simulink model "tcp"  (R2021b)
settings: Solver=VariableStepAuto  StartTime=0.0  StopTime=inf  RelTol=1e-3
undefined symbols (not defined in the file): f
libraries: instrumentlib x4
settings Model: Creator=sdoda3  LastModifiedBy=ae-dagbeyibor3

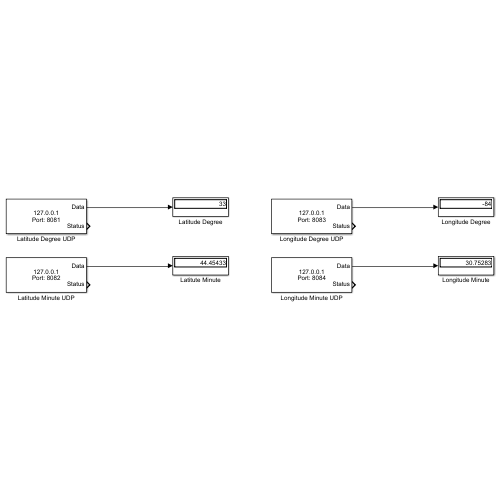
[thumbnail: Simulink's stored preview of the top-level diagram]
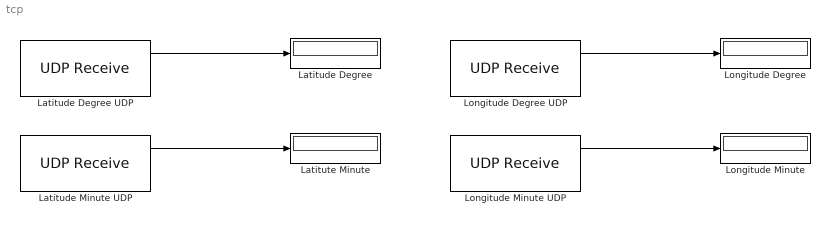
== system tcp ==
  Latitude Degree : Display
  Latitude Degree UDP : instrumentlib/UDP Receive  Priority=1  Host=127.0.0.1  Port=8081  LocalPort=8081  EnablePortSharing=off  GetLatestData=off  DataSize=[1 1]  DataType=int16  ASCIIFormatting=%f,  Terminator=LF  ByteOrder=BigEndian  EnableBlockingMode=off  Timeout=5  SampleTime=0.01  LocalAddress=127.0.0.1
  Latitude Minute UDP : instrumentlib/UDP Receive  Priority=1  Host=127.0.0.1  Port=8081  LocalPort=8082  EnablePortSharing=off  GetLatestData=off  DataSize=[1 1]  DataType=single  ASCIIFormatting=%f,  Terminator=LF  ByteOrder=BigEndian  EnableBlockingMode=off  Timeout=5  SampleTime=0.01  LocalAddress=127.0.0.1
  Latitute Minute : Display
  Longitude Degree : Display
  Longitude Degree UDP : instrumentlib/UDP Receive  Priority=1  Host=127.0.0.1  Port=8081  LocalPort=8083  EnablePortSharing=off  GetLatestData=off  DataSize=[1 1]  DataType=int16  ASCIIFormatting=%f,  Terminator=LF  ByteOrder=BigEndian  EnableBlockingMode=off  Timeout=5  SampleTime=0.01  LocalAddress=127.0.0.1
  Longitude Minute : Display
  Longitude Minute UDP : instrumentlib/UDP Receive  Priority=1  Host=127.0.0.1  Port=8081  LocalPort=8084  EnablePortSharing=off  GetLatestData=off  DataSize=[1 1]  DataType=single  ASCIIFormatting=%f,  Terminator=LF  ByteOrder=BigEndian  EnableBlockingMode=off  Timeout=5  SampleTime=0.01  LocalAddress=127.0.0.1
  wires:
  Latitude Degree UDP/1 -> Latitude Degree/1
  Longitude Degree UDP/1 -> Longitude Degree/1
  Latitude Minute UDP/1 -> Latitute Minute/1
  Longitude Minute UDP/1 -> Longitude Minute/1
